simulink model "model_based_imp_ctrl_R2017a"  (R2017a)
settings: Solver=VariableStepAuto  StartTime=0.0  StopTime=20  FixedStep=0.00040  RelTol=1e-4  AbsTol=1e-7
InitFcn:
  | Parameter
values from neighbouring files (symbols this model uses):
  alpha = pi/180 * 13.6    (= 0.237364778271)    [IdealParameter.m]    (also in ParLuk11.m = deg2rad(13.6); Parameter.m = [-alpha_i;alpha_i;-alpha_i;alpha_i;-alpha_i;alpha_i]; ParameterIdeal.m = [-alpha_i;alpha_i;-alpha_i;alpha_i;-alpha_i;alpha_i]; ParameterVIVE.m = [alpha_i;-alpha_i;alpha_i;-alpha_i;alpha_i;-alpha_i])
  alpha_0 = alpha    (= 0.237364778271)    [IdealParameter.m]    (also in Parameter.m = alpha; ParameterIdeal.m = alpha*1.01; ParameterVIVE.m = alpha*1.01; ParameterVO.m = alpha*1.01)
  angular_noise = 0    [IdealParameter.m]    (also in Parameter.m = 0.5; ParameterIdeal.m; ParameterVIVE.m; ParameterVO.m)
  b = 1.1e-06    [IdealParameter.m]    (also in ParLuk11.m = 1.14e-07; Parameter.m = 8.944e-07; ParameterIdeal.m; ParameterVIVE.m)
  b_0 = b*1.15    (= 1.265e-06)    [IdealParameter.m]    (also in Parameter.m = 8.944e-07; ParameterIdeal.m; ParameterVIVE.m; ParameterVO.m)
  beta = 0    [IdealParameter.m]    (also in ParLuk11.m; Parameter.m = [beta_i; beta_i; beta_i; beta_i; beta_i; beta_i]; ParameterIdeal.m = [beta_i; beta_i; beta_i; beta_i; beta_i; beta_i]; ParameterVIVE.m = [beta_i; beta_i; beta_i; beta_i; beta_i; beta_i])
  beta_0 = beta    (= 0)    [IdealParameter.m]    (also in Parameter.m = beta; ParameterIdeal.m = beta*0.99; ParameterVIVE.m = beta*0.99; ParameterVO.m = beta*0.99)
  deltah = -0.0427    [Parameter.m]    (also in ParameterIdeal.m; ParameterVIVE.m = 0; ParameterVO.m; Parameter_old.m)
  deltah_0 = deltah    (= -0.0427)    [Parameter.m]    (also in ParameterIdeal.m = -0.041419; ParameterVIVE.m = 0; ParameterVO.m = -0.041419; Parameter_old.m = -0.041419)
  eta_rot = 50    [IdealParameter.m]    (also in Parameter.m = 2; ParameterIdeal.m = 20; ParameterVIVE.m = 5; ParameterVO.m = 2)
  g = 9.81    [IdealParameter.m]    (also in ParLuk11.m; Parameter.m; ParameterIdeal.m; ParameterVIVE.m)
  g_0 = g*0.99    (= 9.7119)    [IdealParameter.m]    (also in Parameter.m = 9.81; ParameterIdeal.m = 9.81; ParameterVIVE.m = 9.81; ParameterVO.m = 9.81)
  IB = [Ixx 0 0; 0 Iyy 0; 0 0 Izz]    [IdealParameter.m]    (also in ParLuk11.m; Parameter.m; ParameterIdeal.m; ParameterVIVE.m)
  IB_0 = IB*1.07    [IdealParameter.m]    (also in Parameter.m = IB; ParameterIdeal.m; ParameterVIVE.m; ParameterVO.m)
  Ip = [Ipx 0 0; 0 Ipy 0; 0 0 Ipz]    [Parameter.m]    (also in ParameterIdeal.m; ParameterVIVE.m; ParameterVO.m; Parameter_old.m)
  k = 5.6e-05    [IdealParameter.m]    (also in ParLuk11.m = 2.98e-06; Parameter.m = 4.472e-05; ParameterIdeal.m; ParameterVIVE.m = 5.13e-05)
  K_0 = Ts/(T_rotor_0+Ts)    (= 0.0384615384615)    [IdealParameter.m]    (also in Parameter.m = 0.230769230769; ParameterIdeal.m; ParameterVIVE.m = 0.0350877192982; ParameterVO.m = 0.214285714286)
  k_0 = k*1.16    (= 6.496e-05)    [IdealParameter.m]    (also in Parameter.m = 4.472e-05; ParameterIdeal.m; ParameterVIVE.m = 5.9508e-05; ParameterVO.m)
  K_d_star = 4*eye(3)    [Parameter.m]    (also in ParameterIdeal.m; ParameterVIVE.m; ParameterVO.m; Parameter_old.m)
  K_p_star = 50*eye(3)    [Parameter.m]    (also in ParameterIdeal.m; ParameterVIVE.m; ParameterVO.m; Parameter_old.m)
  L = 0.4    [IdealParameter.m]    (also in ParLuk11.m = 1; Parameter.m; ParameterIdeal.m; ParameterVIVE.m = 0.6)
  L_0 = L*1.02    (= 0.408)    [IdealParameter.m]    (also in Parameter.m = 0.4; ParameterIdeal.m; ParameterVIVE.m = 0.612; ParameterVO.m)
  lambda_rot = 10    [IdealParameter.m]    (also in Parameter.m = 3; ParameterIdeal.m; ParameterVIVE.m = 5; ParameterVO.m = 3)
  m = 1    [Controllability.m]    (also in IdealParameter.m = 2.5; ParLuk11.m = 0.6; Parameter.m = 4.85; ParameterIdeal.m = 4.85)
  m_0 = m*1.03    (= 2.575)    [IdealParameter.m]    (also in Parameter.m = 4.85; ParameterIdeal.m = 4.9955; ParameterVIVE.m = 4.52994; ParameterVO.m = 4.9955)
  M_rot = 50    [IdealParameter.m]    (also in Parameter.m = 6; ParameterIdeal.m = 15; ParameterVIVE.m = 1; ParameterVO.m = 6)
  M_star = m_0*eye(3)    [Parameter.m]    (also in ParameterIdeal.m; ParameterVIVE.m; ParameterVO.m; Parameter_old.m)
  mp = 0.05    [Parameter.m]    (also in ParameterIdeal.m; ParameterVIVE.m; ParameterVO.m; Parameter_old.m)
  omega_noise = 0    [IdealParameter.m]    (also in Parameter.m = sqrt(2)*angular_noise/Ts * pi/180; ParameterIdeal.m; ParameterVIVE.m; ParameterVO.m)
  p_noise = 0    [IdealParameter.m]    (also in Parameter.m = 0.001; ParameterIdeal.m; ParameterVIVE.m; ParameterVO.m)
  T_delay = 0    [IdealParameter.m]    (also in Parameter.m = 0.1; ParameterIdeal.m; ParameterVIVE.m = 0.04; ParameterVO.m = 0.1)
  T_rotor = 0.1    [IdealParameter.m]    (also in Parameter.m; ParameterIdeal.m; ParameterVIVE.m; ParameterVO.m)
  Ts = 1/250    (= 0.004)    [IdealParameter.m]    (also in Parameter.m = 0.03; ParameterIdeal.m; ParameterVIVE.m; ParameterVO.m = 0.03)
  v_noise = 0    [IdealParameter.m]    (also in Parameter.m = sqrt(2)*p_noise/Ts; ParameterIdeal.m; ParameterVIVE.m; ParameterVO.m)
  z_p_0 = T_rotor_0/(T_rotor_0+Ts)    (= 0.961538461538)    [IdealParameter.m]    (also in Parameter.m = 0.769230769231; ParameterIdeal.m; ParameterVIVE.m = 0.964912280702; ParameterVO.m = 0.785714285714)
undefined symbols (not defined in the file or in its folder): DiscIntNeverNeededParam, magnitude, mm
libraries: simulink x7, vrlib x2, slctrlblks x1, dspinverses x1
(part 2 of 3)

== matlab function model_based_imp_ctrl_R2017a/control allocation1/compute nominal effectiveness Matrices/MATLAB Function6 ==
  data: F output; e_r1 input; e_r2 input; e_r3 input; e_r4 input; e_r5 input; e_r6 input; b input; k input; L input; H output
function [F,H]= computeCouplingMatrix(e_r1, e_r2, e_r3, e_r4, e_r5, e_r6, b, k, L)
% u = w^2

F = zeros(3,6);
H = zeros(3,6);

e_r = [e_r1 e_r2 e_r3 e_r4 e_r5 e_r6];

for it = 1:6
    gamma_i = (2*it-3)*pi/6;
   
    % thrust direction
    e_ri = e_r(:,it);
    
    % rotor position vector
    r_Ti =  L * [cos(gamma_i);
            sin(gamma_i);
            0];
        
    % Thrust force
    F(:,it) = k*e_ri;   
    
    % thrust and drag moment
    H(:,it) = k * cross(r_Ti, e_ri) + b * (-1)^it * e_ri;
    
end

== matlab function model_based_imp_ctrl_R2017a/control allocation1/omega_square to omega ==
  data: u input; y output
function y = square2omega(u)

y = sqrt(abs(u)).*sign(u);

== matlab function model_based_imp_ctrl_R2017a/DC Motor Dynamics incl. FF/MATLAB Function2 ==
  data: u input; y output
function y = fcn(u)

y = sqrt(abs(u))*sign(u);

== matlab function model_based_imp_ctrl_R2017a/DC Motor Dynamics incl. FF/MATLAB Function3 ==
  data: u input; y output
function y = fcn(u)

y = u^2*sign(u);

== matlab function model_based_imp_ctrl_R2017a/create Force2 ==
  data: t input; f_ext output
function f_ext = createforce(t)

if t < 10  %15
    %zeros
    %
    f_ext=[0;0;0];
    
elseif (10<t)&&(t<35)
    f_ext=[10;10;10];
    
else
    f_ext=[0;0;0];
    
%     
%         t = t-10;
%     xa = 0;
%     xe = 1;
%     te = 5;
%     x = xa + 10*(xe-xa)*t^3/te^3 - 15*(xe-xa)*t^4/te^4 + 6*(xe-xa)*t^5/te^5;
%     x_dot = 3*10*(xe-xa)*t^2/te^3 - 4*15*(xe-xa)*t^3/te^4 + 5*6*(xe-xa)*t^4/te^5;
%     x_dot_dot = 6*10*(xe-xa)*t/te^3 - 12*15*(xe-xa)*t^2/te^4 + 20*6*(xe-xa)*t^3/te^5;
%     if (t> te)
%         x = xe;
%         x_dot = 0;
%         x_dot_dot = 0;
%     end
%     p_d = [x;0;x];
%     p_d_dot = [x_dot;0;x_dot];
%     p_d_dotdot = [x_dot_dot;0;x_dot_dot];
%     
%     xe = 0.5;
%     x = xa + 10*(xe-xa)*t^3/te^3 - 15*(xe-xa)*t^4/te^4 + 6*(xe-xa)*t^5/te^5;
%     x_dot = 3*10*(xe-xa)*t^2/te^3 - 4*15*(xe-xa)*t^3/te^4 + 5*6*(xe-xa)*t^4/te^5;
%     x_dot_dot = 6*10*(xe-xa)*t/te^3 - 12*15*(xe-xa)*t^2/te^4 + 20*6*(xe-xa)*t^3/te^5;
%     if (t> te)
%         x = xe;
%         x_dot = 0;
%         x_dot_dot = 0;
%     end
%     p_d(3) = x;
%     p_d_dot(3) = x_dot;
%     p_d_dotdot(3) = x_dot_dot;
%     
%     a = 2*pi/te;
%     ct = cos(a*t);
%     st = sin(a*t);
%     
%     R_d = [ct, -st, 0; 
%            st, ct, 0;
%            0 0 1];
%     R_d_dot = [-a*st, -a*ct, 0;
%                 a*ct, -a*st, 0;
%                 0 0 0];
%     R_d_dotdot = [-a*a*ct, a*a*st, 0;
%                    -a*a*st, -a*a*ct, 0;
%                    0 0 0];
%                
%     T_d_tilde = [R_d', -R_d'*p_d; 0,0,0,1]*[R_d_dot p_d_dot; 0,0,0,0];
%     
%     omega_d = skew2vec(T_d_tilde(1:3,1:3));
%     
%     T_d_tilde_dot = [R_d_dot'*R_d_dot+R_d'*R_d_dotdot, R_d_dot'*p_d_dot+R_d'*p_d_dotdot;
%         0,0,0,0];
%     
%     omega_d_dot = skew2vec(T_d_tilde_dot(1:3,1:3));
%     
%     T_D = [omega_d; T_d_tilde(1:3,4)];
%     T_D_dot = [omega_d_dot; T_d_tilde_dot(1:3,4)];
%     
%     if t>te
%         R_d = eye(3);
%         omega_d = [0;0;0];
%         omega_d_dot = [0;0;0];
%         T_D = zeros(6,1);
%         T_D_dot = zeros(6,1);
%     end
end
% 
% p_d = [0;0;0];
%     p_d_dot = [0;0;0];
%     p_d_dotdot = [0;0;0];
%     R_d = eye(3);
%     omega_d = [0;0;0];
%     omega_d_dot = [0;0;0];
%     T_D = zeros(6,1);
%     T_D_dot = zeros(6,1);

== matlab function model_based_imp_ctrl_R2017a/control effectiveness model1/omega to omega_square ==
  data: u input; y output
function y = omega2square(u)

y = u.^2.*sign(u);

== matlab function model_based_imp_ctrl_R2017a/Motion Equations backup/MATLAB Function ==
  data: q input; R output
function R = Quat2R(q)
% compute R from quaternion input

R = [q(1)^2 - q(2)^2 - q(3)^2 + q(4)^2,  2*(q(1)*q(2) - q(3)*q(4)),          2*(q(1)*q(3) + q(2)*q(4));
     2*(q(1)*q(2) + q(3)*q(4)),         -q(1)^2 + q(2)^2 - q(3)^2 + q(4)^2,  2*(q(2)*q(3) - q(1)*q(4));
     2*(q(1)*q(3) - q(2)*q(4)),          2*(q(2)*q(3) + q(1)*q(4)),         -q(1)^2 - q(2)^2 + q(3)^2 + q(4)^2];

== matlab function model_based_imp_ctrl_R2017a/Motion Equations backup/MATLAB Function01 ==
  data: L input; result output; alpha input; deltah input; R_dot input; q input; v_I input
function result = result_deltah(L,alpha,deltah,R_dot,q,v_I)

e_r = zeros(4,6);
result=zeros(4,1);
for it = 1:6
    alpha_i = alpha *(-1)^(it+1);
    gamma_i = (it-1)*pi/3;
    ca = cos(alpha_i);
    sa = sin(alpha_i);
    cy = cos(gamma_i);
    sy = sin(gamma_i);
    
    A = R_dot*[ L*cy+sa*sy*deltah;
        L*sy- sa*cy*deltah;
        ca*deltah];
    A_jacobian_q_dot=[ 2*q(1)*(L*cy + deltah*sa*sy) + 2*q(2)*(L*sy - cy*deltah*sa) + 2*ca*deltah*q(3), 2*q(2)*(L*cy + deltah*sa*sy) - 2*q(1)*(L*sy - cy*deltah*sa) - 2*ca*deltah*q(4), 2*q(3)*(L*cy + deltah*sa*sy) + 2*q(4)*(L*sy - cy*deltah*sa) - 2*ca*deltah*q(1);
        2*q(1)*(L*sy - cy*deltah*sa) - 2*q(2)*(L*cy + deltah*sa*sy) + 2*ca*deltah*q(4), 2*q(1)*(L*cy + deltah*sa*sy) + 2*q(2)*(L*sy - cy*deltah*sa) + 2*ca*deltah*q(3), 2*q(3)*(L*sy - cy*deltah*sa) - 2*q(4)*(L*cy + deltah*sa*sy) - 2*ca*deltah*q(2);
        2*ca*deltah*q(1) - 2*q(4)*(L*sy - cy*deltah*sa) - 2*q(3)*(L*cy + deltah*sa*sy), 2*q(4)*(L*cy + deltah*sa*sy) - 2*q(3)*(L*sy - cy*deltah*sa) + 2*ca*deltah*q(2), 2*q(1)*(L*cy + deltah*sa*sy) + 2*q(4)*(L*sy - cy*deltah*sa) + 2*ca*deltah*q(3);
        2*q(1)*(L*cy + deltah*sa*sy) - 2*q(3)*(L*sy - cy*deltah*sa) + 2*ca*deltah*q(2), 2*q(3)*(L*cy + deltah*sa*sy) + 2*q(4)*(L*sy - cy*deltah*sa) - 2*ca*deltah*q(1), 2*q(1)*(L*sy - cy*deltah*sa) - 2*q(2)*(L*cy + deltah*sa*sy) + 2*ca*deltah*q(4)];
    
    e_r(:,it) =2*A_jacobian_q_dot*(A+v_I);
    result=result+ e_r(:,it);
end

== matlab function model_based_imp_ctrl_R2017a/control effectiveness model1/true control effectiveness matrix/MATLAB Function5 ==
  data: e_r1 output; e_r2 output; e_r3 output; e_r4 output; e_r5 output; e_r6 output; alpha input; beta input
function [e_r1, e_r2, e_r3, e_r4, e_r5, e_r6] = computeThrustDirections(alpha, beta)

e_r = zeros(3,6);
for it = 1:6
    alpha_i = alpha(it);
    beta_i = beta(it);
    gamma_i = (it-1)*pi/3 - pi/6;
    ca = cos(alpha_i);
    sa = sin(alpha_i);
    cb = cos(beta_i);
    sb = sin(beta_i);
    cy = cos(gamma_i);
    sy = sin(gamma_i);
    
    e_r(:,it) = [ca*sb*cy + sa*sy;
                ca*sb*sy - sa*cy;
                ca*cb];
            
end

e_r1 = e_r(:,1);
e_r2 = e_r(:,2);
e_r3 = e_r(:,3);
e_r4 = e_r(:,4);
e_r5 = e_r(:,5);
e_r6 = e_r(:,6);

== matlab function model_based_imp_ctrl_R2017a/control effectiveness model1/true control effectiveness matrix/MATLAB Function6 ==
  data: F output; e_r1 input; e_r2 input; e_r3 input; e_r4 input; e_r5 input; e_r6 input; b input; k input; L input; H output
function [F,H]= computeCouplingMatrix(e_r1, e_r2, e_r3, e_r4, e_r5, e_r6, b, k, L)
% u = w^2

F = zeros(3,6);
H = zeros(3,6);

e_r = [e_r1 e_r2 e_r3 e_r4 e_r5 e_r6];

for it = 1:6
    gamma_i = (2*it-3)*pi/6;
   
    % thrust direction
    e_ri = e_r(:,it);
    
    % rotor position vector
    r_Ti =  L * [cos(gamma_i);
            sin(gamma_i);
            0];
        
    % Thrust force
    F(:,it) = k*e_ri;   
    
    % thrust and drag moment
    H(:,it) = k * cross(r_Ti, e_ri) + b * (-1)^it * e_ri;
    

    
end

== matlab function model_based_imp_ctrl_R2017a/Motion Equations backup/MATLAB Function02 ==
  data: S_trans input; result0 output; alpha input; q_dot input; q input; Ip input; Im input; result1 output
function [result0,result1] = result_deltah(S_trans,alpha,q_dot,q,Ip,Im)

e_r = zeros(4,6);
result0=zeros(4,1);
result1=zeros(4,6);
for it = 1:6
    alpha_i = alpha *(-1)^(it+1);
    gamma_i = (it-1)*pi/3;
    ca = cos(alpha_i);
    sa = sin(alpha_i);
    cy = cos(gamma_i);
    sy = sin(gamma_i);
%     w_m =w_motor(it);
%     B = 4*S_trans*q_dot+[ sa*sy;
%         - sa*cy;
%         ca]*w_m;
    B_jacobian_q_dot=[  2*q(4), -2*q(3),  2*q(2);
  2*q(3),  2*q(4), -2*q(1);
 -2*q(2),  2*q(1),  2*q(4);
 -2*q(1), -2*q(2), -2*q(3)];
    e_r(:,it) =B_jacobian_q_dot*[Ip(1,1)+Im(1,1),0,0;0,Ip(2,2)+Im(2,2),0;0,0,Ip(3,3)+Im(3,3)]*4*S_trans*q_dot;
    result0=result0+ e_r(:,it);
    result1(:,it) =B_jacobian_q_dot*[Ip(1,1)+Im(1,1),0,0;0,Ip(2,2)+Im(2,2),0;0,0,Ip(3,3)+Im(3,3)]*[ sa*sy;- sa*cy;ca];
    
end

== matlab function model_based_imp_ctrl_R2017a/Motion Equations backup/MATLAB Function03 ==
  data: L input; result output; alpha input; R_dot input; q input; v_I input
function result = result_deltah(L,alpha,R_dot,q,v_I)

e_r = zeros(4,6);
result=zeros(4,1);
for it = 1:6
    alpha_i = alpha *(-1)^(it+1);
    gamma_i = (it-1)*pi/3;
    ca = cos(alpha_i);
    sa = sin(alpha_i);
    cy = cos(gamma_i);
    sy = sin(gamma_i);
    
    C = R_dot*[ L*cy;
        L*sy;
        0];
    C_jacobian_q_dot=[   2*L*sy*q(2) + 2*L*cy*q(1), 2*L*cy*q(2) - 2*L*sy*q(1), 2*L*sy*q(4) + 2*L*cy*q(3);
        2*L*sy*q(1) - 2*L*cy*q(2), 2*L*sy*q(2) + 2*L*cy*q(1), 2*L*sy*q(3) - 2*L*cy*q(4);
        - 2*L*sy*q(4) - 2*L*cy*q(3) 2*L*cy*q(4) - 2*L*sy*q(3), 2*L*sy*q(2) + 2*L*cy*q(1);
        2*L*cy*q(4) - 2*L*sy*q(3), 2*L*sy*q(4) + 2*L*cy*q(3), 2*L*sy*q(1) - 2*L*cy*q(2)];
    
    e_r(:,it) =2*C_jacobian_q_dot*(C+v_I);
    result=result+ e_r(:,it);
end

== matlab function model_based_imp_ctrl_R2017a/Motion Equations backup/MATLAB Function04 ==
  data: L input; result output; alpha input; deltah input; R_dot input; q_dot input; v_I input
function result = result_deltah(L,alpha,deltah,R_dot,q_dot,v_I)

e_r = zeros(4,6);
result=zeros(4,1);
for it = 1:6
    alpha_i = alpha *(-1)^(it+1);
    gamma_i = (it-1)*pi/3;
    ca = cos(alpha_i);
    sa = sin(alpha_i);
    cy = cos(gamma_i);
    sy = sin(gamma_i);
    
    A = R_dot*[ L*cy+sa*sy*deltah;
        L*sy- sa*cy*deltah;
        ca*deltah];
    A_jacobian_q= [ 2*q_dot(1)*(L*cy + deltah*sa*sy) + 2*q_dot(2)*(L*sy - cy*deltah*sa) + 2*ca*deltah*q_dot(3), 2*q_dot(2)*(L*cy + deltah*sa*sy) - 2*q_dot(1)*(L*sy - cy*deltah*sa) - 2*ca*deltah*q_dot(4), 2*q_dot(3)*(L*cy + deltah*sa*sy) + 2*q_dot(4)*(L*sy - cy*deltah*sa) - 2*ca*deltah*q_dot(1);
        2*q_dot(1)*(L*sy - cy*deltah*sa) - 2*q_dot(2)*(L*cy + deltah*sa*sy) + 2*ca*deltah*q_dot(4), 2*q_dot(1)*(L*cy + deltah*sa*sy) + 2*q_dot(2)*(L*sy - cy*deltah*sa) + 2*ca*deltah*q_dot(3), 2*q_dot(3)*(L*sy - cy*deltah*sa) - 2*q_dot(4)*(L*cy + deltah*sa*sy) - 2*ca*deltah*q_dot(2);
        2*ca*deltah*q_dot(1) - 2*q_dot(4)*(L*sy - cy*deltah*sa) - 2*q_dot(3)*(L*cy + deltah*sa*sy), 2*q_dot(4)*(L*cy + deltah*sa*sy) - 2*q_dot(3)*(L*sy - cy*deltah*sa) + 2*ca*deltah*q_dot(2), 2*q_dot(1)*(L*cy + deltah*sa*sy) + 2*q_dot(2)*(L*sy - cy*deltah*sa) + 2*ca*deltah*q_dot(3);
        2*q_dot(4)*(L*cy + deltah*sa*sy) - 2*q_dot(3)*(L*sy - cy*deltah*sa) + 2*ca*deltah*q_dot(2), 2*q_dot(3)*(L*cy + deltah*sa*sy) + 2*q_dot(4)*(L*sy - cy*deltah*sa) - 2*ca*deltah*q_dot(1), 2*q_dot(1)*(L*sy - cy*deltah*sa) - 2*q_dot(2)*(L*cy + deltah*sa*sy) + 2*ca*deltah*q_dot(4)];
    
    e_r(:,it) =2*A_jacobian_q*(A+v_I);
    result=result+ e_r(:,it);
end

== matlab function model_based_imp_ctrl_R2017a/Motion Equations backup/MATLAB Function05 ==
  data: S_trans input; result0 output; alpha input; q_dot input; Ip input; Im input; result1 output
function [result0,result1] = result_deltah(S_trans,alpha,q_dot,Ip,Im)

e_r = zeros(4,6);
result0=zeros(4,1);
result1=zeros(4,6);
for it = 1:6
    alpha_i = alpha *(-1)^(it+1);
    gamma_i = (it-1)*pi/3;
    ca = cos(alpha_i);
    sa = sin(alpha_i);
    cy = cos(gamma_i);
    sy = sin(gamma_i);
    %     w_m =w_motor(it);
    %     B = 4*S_trans*q_dot+[ sa*sy;
    %         - sa*cy;
    %         ca]*w_m;
    B_jacobian_q=[ -2*q_dot(4),  2*q_dot(3), -2*q_dot(2);
        -2*q_dot(3), -2*q_dot(4),  2*q_dot(4);
        2*q_dot(2), -2*q_dot(1), -2*q_dot(4);
        2*q_dot(1),  2*q_dot(2),  2*q_dot(3)];
    e_r(:,it) =B_jacobian_q*[Ip(1,1)+Im(1,1),0,0;0,Ip(2,2)+Im(2,2),0;0,0,Ip(3,3)+Im(3,3)]*4*S_trans*q_dot;
    result0=result0+ e_r(:,it);
    result1(:,it) =B_jacobian_q*[Ip(1,1)+Im(1,1),0,0;0,Ip(2,2)+Im(2,2),0;0,0,Ip(3,3)+Im(3,3)]*[ sa*sy;- sa*cy;ca];
end

== matlab function model_based_imp_ctrl_R2017a/Motion Equations backup/MATLAB Function06 ==
  data: L input; result output; alpha input; R_dot input; q_dot input; v_I input
function result = result_deltah(L,alpha,R_dot,q_dot,v_I)

e_r = zeros(4,6);
result=zeros(4,1);
for it = 1:6
    alpha_i = alpha *(-1)^(it+1);
    gamma_i = (it-1)*pi/3;
    ca = cos(alpha_i);
    sa = sin(alpha_i);
    cy = cos(gamma_i);
    sy = sin(gamma_i);
    
    C = R_dot*[ L*cy;
        L*sy;
        0];
    C_jacobian_q_dot=[   2*L*cy*q_dot(1) + 2*L*q_dot(2)*sy, 2*L*cy*q_dot(2) - 2*L*q_dot(1)*sy, 2*L*cy*q_dot(3) + 2*L*q_dot(4)*sy;
        2*L*q_dot(1)*sy - 2*L*cy*q_dot(2), 2*L*cy*q_dot(1) + 2*L*q_dot(2)*sy, 2*L*q_dot(3)*sy - 2*L*cy*q_dot(4);
        - 2*L*cy*q_dot(3) - 2*L*q_dot(4)*sy, 2*L*cy*q_dot(4) - 2*L*q_dot(3)*sy, 2*L*cy*q_dot(1) + 2*L*q_dot(2)*sy;
        2*L*cy*q_dot(4) - 2*L*q_dot(3)*sy, 2*L*cy*q_dot(3) + 2*L*q_dot(4)*sy, 2*L*q_dot(1)*sy - 2*L*cy*q_dot(2)];
    
    e_r(:,it) =2*C_jacobian_q_dot*(C+v_I);
    result=result+ e_r(:,it);
end

== matlab function model_based_imp_ctrl_R2017a/Motion Equations backup/MATLAB Function07 ==
  data: alpha input; deltah input; q input; result output
function result = result_deltah(alpha,deltah,q)

e_r = zeros(4,6);
result=zeros(4,1);
for it = 1:6
    alpha_i = alpha *(-1)^(it+1);
    gamma_i = (it-1)*pi/3;
    ca = cos(alpha_i);
    sa = sin(alpha_i);
    cy = cos(gamma_i);
    sy = sin(gamma_i);
    
    M4=2*[-q(2),-q(1),q(4);q(3),-q(4),-q(1);-q(4),-q(3),-q(2);q(1),-q(2),q(3)];
    e_r(:,it) = M4*[ sa*sy*deltah;
        sa*cy*deltah;
        ca*deltah];
    result=result+ e_r(:,it);
end

== matlab function model_based_imp_ctrl_R2017a/Motion Equations backup/MATLAB Function1 ==
  data: w input; Q output
function Q = omegaSkew(w)
%#codegen

Q = [0 w(3) -w(2) w(1);
    -w(3) 0 w(1) w(2);
    w(2) -w(1) 0 w(3);
    -w(1) -w(2) -w(3) 0];

== matlab function model_based_imp_ctrl_R2017a/Motion Equations backup/MATLAB Function10 ==
  data: factor1 input; add_result output; factor2 input
function add_result = addition(factor1,factor2)

add_result = factor1+factor2;

== matlab function model_based_imp_ctrl_R2017a/combination of Imp and slid_Control/MATLAB Function1 ==
  data: R input; q output
function q   = DCM2Quat(R)

%%%%%%%%%%%%%%%%%%%%%%%%%%%%%%%%%%%%%%%%%%%%%%%%%%%%%%%%%%%%%%%%%%%%%%%%%%%
%
% M-file: Tool_DCM2Quat
%         -> impelmeted as M-Function
% Author: Marcel Tkocz
% Version: 27.01.2008
%
% Description:
%   This Function converts roll-pitch-yaw angels into their quaternion
%   equivalents.
%
% Inputs:
%   Orientation ... orientation in roll-pitch-yaw angels
%
% Outputs:
%   q           ... orientation in quaternions
%   
%%%%%%%%%%%%%%%%%%%%%%%%%%%%%%%%%%%%%%%%%%%%%%%%%%%%%%%%%%%%%%%%%%%%%%%%%%%

%--------------------------------------------------------------------------
% Calculation of Quaternions based on q1
%--------------------------------------------------------------------------
q = [0 0 0 1]';

if (1 + R(1,1) - R(2,2) - R(3,3)) > 0 
    q1 = 1/2*sqrt(1 + R(1,1) - R(2,2) - R(3,3));
    q2 = 1/(4*q1)*( R(1,2) + R(2,1));
    q3 = 1/(4*q1)*( R(1,3) + R(3,1));
    q4 = 1/(4*q1)*(-R(2,3) + R(3,2));

    if round(q1) ~= 0
        q = [q1; q2; q3; q4];
    end
end

%--------------------------------------------------------------------------
% Calculation of Quaternions based on q2
%--------------------------------------------------------------------------

if (1 - R(1,1) + R(2,2) - R(3,3)) > 0
    q2 = 1/2*sqrt(1 - R(1,1) + R(2,2) - R(3,3));
    q1 = 1/(4*q2)*( R(1,2) + R(2,1));
    q3 = 1/(4*q2)*( R(2,3) + R(3,2));
    q4 = 1/(4*q2)*( R(1,3) - R(3,1));

    if round(q2) ~= 0
        q = [q1; q2; q3; q4];
    end
end

%--------------------------------------------------------------------------
% Calculation of Quaternions based on q3
%--------------------------------------------------------------------------

if (1 - R(1,1) - R(2,2) + R(3,3)) > 0
    q3 = 1/2*sqrt(1 - R(1,1) - R(2,2) + R(3,3));
    q1 = 1/(4*q3)*( R(1,3) + R(3,1));
    q2 = 1/(4*q3)*( R(2,3) + R(3,2));
    q4 = 1/(4*q3)*(-R(1,2) + R(2,1));

    if round(q3) ~= 0
        q = [q1; q2; q3; q4];
    end
end

%--------------------------------------------------------------------------
% Calculation of Quaternions based on q4
%--------------------------------------------------------------------------

if (1 + R(1,1) + R(2,2) + R(3,3)) > 0
    q4 = 1/2*sqrt(1 + R(1,1) + R(2,2) + R(3,3));
    q1 = 1/(4*q4)*(-R(2,3) + R(3,2));
    q2 = 1/(4*q4)*(-R(3,1) + R(1,3));
    q3 = 1/(4*q4)*(-R(1,2) + R(2,1));

    if round(q4) ~= 0
        q = [q1; q2; q3; q4];
    end
end


end

== matlab function model_based_imp_ctrl_R2017a/combination of Imp and slid_Control/MATLAB Function10 ==
  data: eps_tilde input; G_dot output; eta_tilde input; omega_tilde input
function G_dot = compute_G_dot(eps_tilde, eta_tilde, omega_tilde)

eta_dot = -0.5*eps_tilde'*omega_tilde;

eps_dot = 0.5*(eta_tilde*eye(3) + vec2skew(eps_tilde))*omega_tilde;

if eta_tilde >= 0
    sig = 1;
else
    sig = -1;
end

G_dot = [sig*eps_dot';
        eta_dot*eye(3) + vec2skew(eps_dot)]';

== matlab function model_based_imp_ctrl_R2017a/combination of Imp and slid_Control/MATLAB Function11 ==
  data: s input; u output; z2 input; lambda input; G input; G_dot input; omega_tilde input; omega_d_dot input; omega_B input; IBB input; eta input
function u = compute_u(s,z2,lambda,G,G_dot,omega_tilde,omega_d_dot,omega_B,IBB,eta)

sgn = zeros(4,1);
% avoid chattering
% linear function
for it=1:4
%     if s(it) < 1 && s(it) > -1
%         sgn(it) = s(it);
%     else
%         sgn(it) = sign(s(it));
%     end
    sgn(it) = 2/pi*atan(s(it));
end

u = IBB*G* ( -2*eta*sgn - 2*lambda*z2 - G_dot.'*omega_tilde ) ...
    + IBB*omega_d_dot + cross(omega_B,IBB*omega_B);

== matlab function model_based_imp_ctrl_R2017a/Motion Equations backup/MATLAB Function11 ==
  data: factor1 input; add_result output; factor2 input
function add_result = addition(factor1,factor2)

add_result = factor1+factor2;

== matlab function model_based_imp_ctrl_R2017a/Motion Equations backup/MATLAB Function13 ==
  data: factor1 input; add_result output; factor2 input
function add_result = addition(factor1,factor2)

add_result = factor1+factor2;

== matlab function model_based_imp_ctrl_R2017a/combination of Imp and slid_Control/MATLAB Function14 ==
  data: s_0 input; int_arg output; eta input
function int_arg = computeIntArg(s_0,eta)

sgn = 2/pi*atan(s_0);
int_arg = - eta*sgn;

== matlab function model_based_imp_ctrl_R2017a/Motion Equations backup/MATLAB Function14 ==
  data: omega input; w_x output
function w_x = omegaSkew3D(omega)

w_x = [0 -omega(3) omega(2);
        omega(3) 0 -omega(1);
        -omega(2) omega(1) 0];

== matlab function model_based_imp_ctrl_R2017a/combination of Imp and slid_Control/MATLAB Function15 ==
  data: s input; G input; IB input; u1 output; M input
function u1 = computeU1(s,G,IB,M)


D = 0.5*G.'*inv(IB);
u1 = -M*2/pi*atan(D.'*s);%./norm(D.'*s,2);

== matlab function model_based_imp_ctrl_R2017a/combination of Imp and slid_Control/MATLAB Function2 ==
  data: I input; I_inv output
function I_inv = inverse(I)

I_inv = inv(I);

== matlab function model_based_imp_ctrl_R2017a/combination of Imp and slid_Control/MATLAB Function3 ==
  data: epsilon_d input; eta_d input; epsilon input; eta input; eta_tilde output; epsilon_tilde output; epsilon_tilde_T output; skew_eps_tilde output
function [eta_tilde, epsilon_tilde, epsilon_tilde_T, skew_eps_tilde] = calc_q_tilde(epsilon_d, eta_d, epsilon, eta)

eta_tilde = eta_d*eta + epsilon_d'*epsilon;

epsilon_tilde = -eta * epsilon_d + eta_d*epsilon - vec2skew(epsilon_d)*epsilon;

epsilon_tilde_T = epsilon_tilde';

skew_eps_tilde = vec2skew(epsilon_tilde);

== matlab function model_based_imp_ctrl_R2017a/combination of Imp and slid_Control/MATLAB Function4 ==
  data: eta_tilde input; z1 output; eps_tilde input
function z1 = compute_z1(eta_tilde, eps_tilde)

z1 = [1-abs(eta_tilde);
    eps_tilde];

== matlab function model_based_imp_ctrl_R2017a/Motion Equations backup/MATLAB Function2 ==
  data: S input; S_Trans output
function S_Trans = Trans(S)

S_Trans = S.';

== matlab function model_based_imp_ctrl_R2017a/Motion Equations backup/MATLAB Function3 ==
  data: result output; alpha input; beta input; deltah input; l input
function result = sum_prop_pos(alpha,beta,deltah,l)

% pi_in_B = zeros(3,6);
result=zeros(3,1);
for it = 1:6
%     alpha_i = alpha *(-1)^(it+1);
    gamma_i = (2*it-3)*pi/6;
    ca = cos(alpha(it));
    sa = sin(alpha(it));
    cb = cos(beta(it));
    sb = sin(beta(it));
    cy = cos(gamma_i);
    sy = sin(gamma_i);
    
%     pi_in_B(:,it) = [deltah*(ca*sb*cy + sa*sy) + l*cy;
%                  deltah*(ca*sb*sy - sa*cy) + l*sy;
%                  deltah*ca*cb];
%     
%     result=result+ pi_in_B(:,it);      

    result = result + [ deltah*(ca*sb*cy + sa*sy) + l*cy;...
                        deltah*(ca*sb*sy - sa*cy) + l*sy;...
                        deltah*ca*cb];...
end

== matlab function model_based_imp_ctrl_R2017a/combination of Imp and slid_Control/MATLAB Function7 ==
  data: R input; q output
function q   = DCM2Quat(R)

%%%%%%%%%%%%%%%%%%%%%%%%%%%%%%%%%%%%%%%%%%%%%%%%%%%%%%%%%%%%%%%%%%%%%%%%%%%
%
% M-file: Tool_DCM2Quat
%         -> impelmeted as M-Function
% Author: Marcel Tkocz
% Version: 27.01.2008
%
% Description:
%   This Function converts roll-pitch-yaw angels into their quaternion
%   equivalents.
%
% Inputs:
%   Orientation ... orientation in roll-pitch-yaw angels
%
% Outputs:
%   q           ... orientation in quaternions
%   
%%%%%%%%%%%%%%%%%%%%%%%%%%%%%%%%%%%%%%%%%%%%%%%%%%%%%%%%%%%%%%%%%%%%%%%%%%%

%--------------------------------------------------------------------------
% Calculation of Quaternions based on q1
%--------------------------------------------------------------------------
q = [0 0 0 1]';

if (1 + R(1,1) - R(2,2) - R(3,3)) > 0 
    q1 = 1/2*sqrt(1 + R(1,1) - R(2,2) - R(3,3));
    q2 = 1/(4*q1)*( R(1,2) + R(2,1));
    q3 = 1/(4*q1)*( R(1,3) + R(3,1));
    q4 = 1/(4*q1)*(-R(2,3) + R(3,2));

    if round(q1) ~= 0
        q = [q1; q2; q3; q4];
    end
end

%--------------------------------------------------------------------------
% Calculation of Quaternions based on q2
%--------------------------------------------------------------------------

if (1 - R(1,1) + R(2,2) - R(3,3)) > 0
    q2 = 1/2*sqrt(1 - R(1,1) + R(2,2) - R(3,3));
    q1 = 1/(4*q2)*( R(1,2) + R(2,1));
    q3 = 1/(4*q2)*( R(2,3) + R(3,2));
    q4 = 1/(4*q2)*( R(1,3) - R(3,1));

    if round(q2) ~= 0
        q = [q1; q2; q3; q4];
    end
end

%--------------------------------------------------------------------------
% Calculation of Quaternions based on q3
%--------------------------------------------------------------------------

if (1 - R(1,1) - R(2,2) + R(3,3)) > 0
    q3 = 1/2*sqrt(1 - R(1,1) - R(2,2) + R(3,3));
    q1 = 1/(4*q3)*( R(1,3) + R(3,1));
    q2 = 1/(4*q3)*( R(2,3) + R(3,2));
    q4 = 1/(4*q3)*(-R(1,2) + R(2,1));

    if round(q3) ~= 0
        q = [q1; q2; q3; q4];
    end
end

%--------------------------------------------------------------------------
% Calculation of Quaternions based on q4
%--------------------------------------------------------------------------

if (1 + R(1,1) + R(2,2) + R(3,3)) > 0
    q4 = 1/2*sqrt(1 + R(1,1) + R(2,2) + R(3,3));
    q1 = 1/(4*q4)*(-R(2,3) + R(3,2));
    q2 = 1/(4*q4)*(-R(3,1) + R(1,3));
    q3 = 1/(4*q4)*(-R(1,2) + R(2,1));

    if round(q4) ~= 0
        q = [q1; q2; q3; q4];
    end
end


end

== matlab function model_based_imp_ctrl_R2017a/combination of Imp and slid_Control/MATLAB Function8 ==
  data: eta_tilde input; G output; eps_tilde input
function G = compute_G(eta_tilde, eps_tilde)

if (eta_tilde >= 0)
    sig = 1;
else
    sig = -1;
end

G = [sig*eps_tilde';
    eye(3)*eta_tilde + vec2skew(eps_tilde)]';

== matlab function model_based_imp_ctrl_R2017a/combination of Imp and slid_Control/MATLAB Function9 ==
  data: G input; z2 output; omega_tilde input
function z2 = compute_z2(G,omega_tilde)

z2 = 0.5*G.'*omega_tilde;

== matlab function model_based_imp_ctrl_R2017a/create Force ==
  data: t input; f_ext output
function f_ext = createforce(t)

if (5<t)&&(t<30)
    f_ext=[10;10;10];
    
else
    f_ext=[0;0;0];
    
end
end

== matlab function model_based_imp_ctrl_R2017a/Motion Equations backup/MATLAB Function4 ==
  data: q_dot input; S_dot output
function S_dot= S_dot(q_dot)
% compute R from quaternion input
% tmp_mat =[q(1),q1(t);
%     q(2),q2(t);
%     q(3),q3(t);
%     q(4),q4(t);];

S_dot = 1/2*[ q_dot(4), -q_dot(3), q_dot(2);
    q_dot(3), q_dot(4), -q_dot(1);
    -q_dot(2),q_dot(1),q_dot(4);
    -q_dot(1),-q_dot(2),-q_dot(3)];
%dot_S=diff(S);
% S=subs(S,tmp_mat(:,1),tmp_mat(:,2));

== matlab function model_based_imp_ctrl_R2017a/Motion Equations backup/MATLAB Function5 ==
  data: omega input; w_x output
function w_x = omegaSkew3D(omega)

w_x = [0 -omega(3) omega(2);
        omega(3) 0 -omega(1);
        -omega(2) omega(1) 0];

== matlab function model_based_imp_ctrl_R2017a/Motion Equations backup/MATLAB Function6 ==
  data: q input; S output
function S= Convertfrom(q)
% compute R from quaternion input
% tmp_mat =[q(1),q1(t);
%     q(2),q2(t);
%     q(3),q3(t);
%     q(4),q4(t);];

S = 1/2*[ q(4), -q(3), q(2);
    q(3), q(4), -q(1);
    -q(2),q(1),q(4);
    -q(1),-q(2),-q(3)];
%dot_S=diff(S);
% S=subs(S,tmp_mat(:,1),tmp_mat(:,2));

== matlab function model_based_imp_ctrl_R2017a/Motion Equations backup/MATLAB Function7 ==
  data: S input; S_Trans output
function S_Trans = Trans(S)

S_Trans = S.';
